simulink model "SystemModel"  (Simulink 8.6)
settings: Solver=ode45  StartTime=0.0  StopTime=25  RelTol=1e-3
undefined symbols (not defined in the file): Alt, altSaturation, ControlDriverGain, CurrentDriverBias, mBackEMF, mDrag, mElecDynDen, mElecDynNum, mHeliDynDen, mHeliDynNum, mLiftTorque, mMechDynDen, mMechDynNum, mPID, mSat, mTConst, potentiometerBias, potentiometerGain, RadPerDeg, tBackEMF, tElecDynDen, tElecDynNum, tHeliDynDen, tHeliDynNum, tMechDynDen, tMechDynNum, torqueFromAltMotorMass, torqueFromYawMotorMass, tPID, tSat, tTConst, tTorque, Yaw, yawSaturation
libraries: simulink x4, simulink_extras x1
settings Model: Creator=Leos  LastModifiedBy=Wyatt
settings DataIOCC: LimitDataPoints=off
settings DebuggingCC: ParameterTunabilityLossMsg=error  FcnCallInpInsideContextMsg=UseLocalSettings
settings ConfigComp: CovSFcnEnable=off

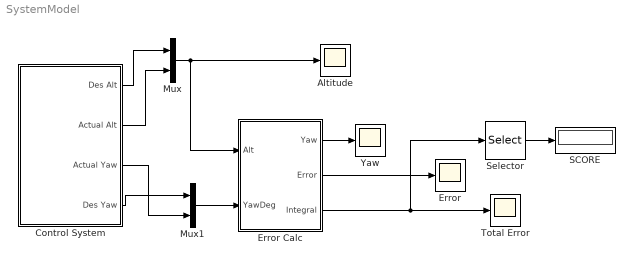
== system SystemModel ==
  Altitude : Scope
  Control System : Subsystem
  Error : Scope
  Error Calc : Subsystem
  Mux : Mux  Inputs=2
  Mux1 : Mux  Inputs=2
  SCORE : Display
  Selector : Selector  InputPortWidth=3  IndexOptions=Index vector (dialog)  Indices=[3]  OutputSizes=1
  Total Error : Scope
  Yaw : Scope
  wires:
  Mux/1 -> Error Calc/1(Alt), Altitude/1
  Control System/1(Des Alt) -> Mux/1
  Control System/2(Actual Alt) -> Mux/2
  Control System/3(Actual Yaw) -> Mux1/2
  Control System/4(Des Yaw) -> Mux1/1
  Mux1/1 -> Error Calc/2(YawDeg)
  Error Calc/1(Yaw) -> Yaw/1
  Error Calc/2(Error) -> Error/1
  Error Calc/3(Integral) -> Selector/1, Total Error/1
  Selector/1 -> SCORE/1

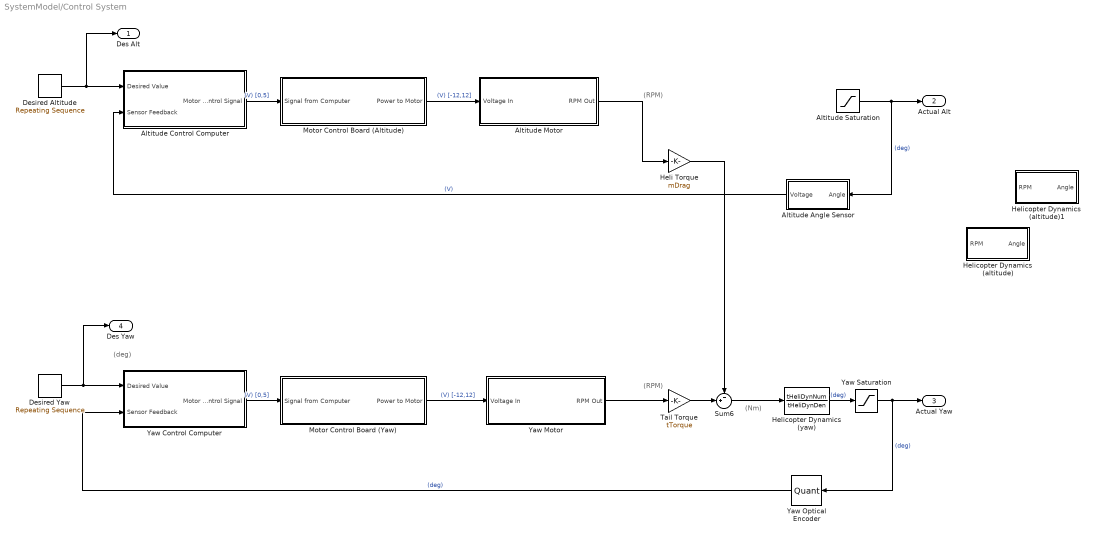
== system SystemModel/Control System ==
  note: (RPM)
  note: (deg)
  note: (RPM)
  note: (Nm)
  Altitude Saturation : Saturate  UpperLimit=altSaturation  LowerLimit=-altSaturation
  Altitude Angle Sensor : Subsystem
  Altitude Control Computer : Subsystem
  Altitude Motor : Subsystem
  Desired Altitude : simulink/Sources/Repeating Sequence  rep_seq_t=Alt(2,:)  rep_seq_y=Alt(1,:)
  Desired Yaw : simulink/Sources/Repeating Sequence  rep_seq_t=Yaw(2,:)  rep_seq_y=Yaw(1,:)
  Heli Torque : Gain  Gain=mDrag
  Helicopter Dynamics (yaw) : TransferFcn  Numerator=tHeliDynNum  Denominator=tHeliDynDen
  Helicopter Dynamics (altitude) : Subsystem
  Helicopter Dynamics (altitude)1 : Subsystem
  Motor Control Board (Altitude) : Subsystem
  Motor Control Board (Yaw) : Subsystem
  Sum6 : Sum  Inputs=-+|
  Tail Torque : Gain  Gain=tTorque
  Yaw Saturation : Saturate  UpperLimit=yawSaturation  LowerLimit=0
  Yaw Control Computer : Subsystem
  Yaw Motor : Subsystem
  Yaw Optical Encoder : Quantizer  QuantizationInterval=yawEncoderQuantization
  Des Alt : Outport
  Actual Alt : Outport  Port=2
  Actual Yaw : Outport  Port=3
  Des Yaw : Outport  Port=4
  wires:
  Desired Altitude/1 -> Altitude Control Computer/1(Desired Value), Des Alt/1
  Helicopter Dynamics (yaw)/1 -> Yaw Saturation/1  "(deg)"
  Desired Yaw/1 -> Yaw Control Computer/1(Desired Value), Des Yaw/1
  Altitude Motor/1(RPM Out) -> Heli Torque/1
  Yaw Optical Encoder/1 -> Yaw Control Computer/2(Sensor Feedback)  "(deg)"
  Yaw Control Computer/1(Motor Driver Control Signal) -> Motor Control Board (Yaw)/1(Signal from Computer)  "(V) [0,5]"
  Altitude Control Computer/1(Motor Driver Control Signal) -> Motor Control Board (Altitude)/1(Signal from Computer)  "(V) [0,5]"
  Motor Control Board (Altitude)/1(Power to Motor) -> Altitude Motor/1(Voltage In)  "(V) [-12,12]"
  Motor Control Board (Yaw)/1(Power to Motor) -> Yaw Motor/1(Voltage In)  "(V) [-12,12]"
  Yaw Motor/1(RPM Out) -> Tail Torque/1
  Altitude Angle Sensor/1(Voltage) -> Altitude Control Computer/2(Sensor Feedback)  "(V)"
  Altitude Saturation/1 -> Actual Alt/1, Altitude Angle Sensor/1(Angle)  "(deg)"
  Yaw Saturation/1 -> Yaw Optical Encoder/1, Actual Yaw/1  "(deg)"
  Tail Torque/1 -> Sum6/2
  Sum6/1 -> Helicopter Dynamics (yaw)/1
  Heli Torque/1 -> Sum6/1

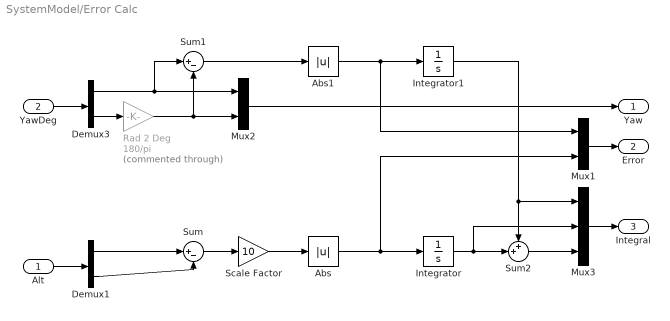
== system SystemModel/Error Calc ==
  Alt : Inport
  YawDeg : Inport  Port=2
  Abs : Abs
  Abs1 : Abs
  Demux1 : Demux  Outputs=2
  Demux3 : Demux  Outputs=2
  Integrator : Integrator
  Integrator1 : Integrator
  Mux1 : Mux  Inputs=2
  Mux2 : Mux  Inputs=2
  Mux3 : Mux  Inputs=3
  Rad 2 Deg : Gain  Commented=through  Gain=180/pi
  Scale Factor : Gain  Gain=10
  Sum : Sum  Inputs=|+-
  Sum1 : Sum  Inputs=|+-
  Sum2 : Sum  Inputs=++|
  Yaw : Outport
  Error : Outport  Port=2
  Integral : Outport  Port=3
  wires:
  YawDeg/1 -> Demux3/1
  Alt/1 -> Demux1/1
  Mux2/1 -> Yaw/1
  Rad 2 Deg/1 -> Sum1/2, Mux2/2
  Demux3/2 -> Rad 2 Deg/1
  Demux3/1 -> Sum1/1, Mux2/1
  Demux1/1 -> Sum/1
  Demux1/2 -> Sum/2
  Sum/1 -> Scale Factor/1
  Mux1/1 -> Error/1
  Sum1/1 -> Abs1/1
  Abs1/1 -> Mux1/1, Integrator1/1
  Scale Factor/1 -> Abs/1
  Abs/1 -> Mux1/2, Integrator/1
  Mux3/1 -> Integral/1
  Integrator/1 -> Mux3/2, Sum2/2
  Integrator1/1 -> Mux3/1, Sum2/1
  Sum2/1 -> Mux3/3

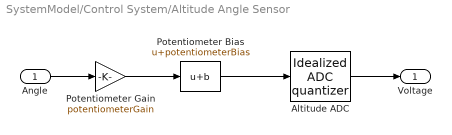
== system SystemModel/Control System/Altitude Angle Sensor ==
  Angle : Inport
  Altitude ADC : simulink_extras/Additional Discrete/Idealized ADC quantizer  NumberOfConverterBits=ADC_bitwidth  Vmin=ground  Vmax=Vss  OutputDataType=int16  OutputNegativeValues=off
  Potentiometer Bias : Bias  Bias=potentiometerBias
  Potentiometer Gain : Gain  Gain=potentiometerGain
  Voltage : Outport
  wires:
  Potentiometer Bias/1 -> Altitude ADC/1
  Angle/1 -> Potentiometer Gain/1
  Potentiometer Gain/1 -> Potentiometer Bias/1
  Altitude ADC/1 -> Voltage/1

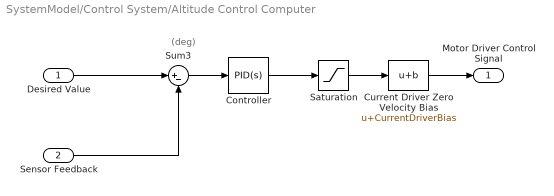
== system SystemModel/Control System/Altitude Control Computer ==
  note: (deg)
  Desired Value : Inport
  Sensor Feedback : Inport  Port=2
  Controller : simulink/Continuous/PID Controller  Controller=PID  TimeDomain=Continuous-time  SampleTime=-1  IntegratorMethod=Forward Euler  FilterMethod=Forward Euler  Form=Parallel  UseFilter=on  ControllerParametersSource=internal  P=mPID(1)  I=mPID(2)  D=mPID(3)  N=100  InitialConditionSource=internal  InitialConditionForIntegrator=0  InitialConditionForFilter=0  ExternalReset=none  LimitOutput=off  UpperSaturationLimit=inf  LowerSaturationLimit=-inf  LinearizeAsGain=on  AntiWindupMode=none  Kb=1  TrackingMode=off  Kt=1  PParamMin=[]  PParamMax=[]  IParamMin=[]  IParamMax=[]  DParamMin=[]  DParamMax=[]  NParamMin=[]  NParamMax=[]  KbParamMin=[]  KbParamMax=[]  KtParamMin=[]  KtParamMax=[]  POutMin=[]  POutMax=[]  IOutMin=[]  IOutMax=[]  DOutMin=[]  DOutMax=[]  NOutMin=[]  NOutMax=[]  KbOutMin=[]  KbOutMax=[]  KtOutMin=[]  KtOutMax=[]  IntegratorOutMin=[]  IntegratorOutMax=[]  FilterOutMin=[]  FilterOutMax=[]  SumOutMin=[]  SumOutMax=[]  SumI1OutMin=[]  SumI1OutMax=[]  SumI2OutMin=[]  SumI2OutMax=[]  SumI3OutMin=[]  SumI3OutMax=[]  SumDOutMin=[]  SumDOutMax=[]  SaturationOutMin=[]  SaturationOutMax=[]  IntegratorContinuousStateAttributes=''  IntegratorStateMustResolveToSignalObject=off  IntegratorRTWStateStorageClass=Auto  FilterContinuousStateAttributes=''  FilterStateMustResolveToSignalObject=off  FilterRTWStateStorageClass=Auto  DifferentiatorICPrevScaledInput=0  DifferentiatorOutMin=[]  DifferentiatorOutMax=[]
  Current Driver Zero Velocity Bias : Bias  Bias=CurrentDriverBias
  Saturation : Saturate  UpperLimit=mSat  LowerLimit=-mSat
  Sum3 : Sum  Inputs=|+-
  Motor Driver Control Signal : Outport
  wires:
  Desired Value/1 -> Sum3/1
  Sensor Feedback/1 -> Sum3/2
  Sum3/1 -> Controller/1
  Saturation/1 -> Current Driver Zero Velocity Bias/1
  Controller/1 -> Saturation/1
  Current Driver Zero Velocity Bias/1 -> Motor Driver Control Signal/1

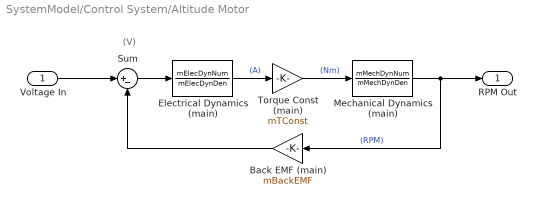
== system SystemModel/Control System/Altitude Motor ==
  note: (V)
  Voltage In : Inport
  Back EMF (main) : Gain  Gain=mBackEMF
  Electrical Dynamics (main) : TransferFcn  Numerator=mElecDynNum  Denominator=mElecDynDen
  Mechanical Dynamics (main) : TransferFcn  Numerator=mMechDynNum  Denominator=mMechDynDen
  Sum : Sum  Inputs=|+-
  Torque Const (main) : Gain  Gain=mTConst
  RPM Out : Outport
  wires:
  Voltage In/1 -> Sum/1
  Torque Const (main)/1 -> Mechanical Dynamics (main)/1  "(Nm)"
  Back EMF (main)/1 -> Sum/2
  Mechanical Dynamics (main)/1 -> RPM Out/1, Back EMF (main)/1  "(RPM)"
  Electrical Dynamics (main)/1 -> Torque Const (main)/1  "(A)"
  Sum/1 -> Electrical Dynamics (main)/1

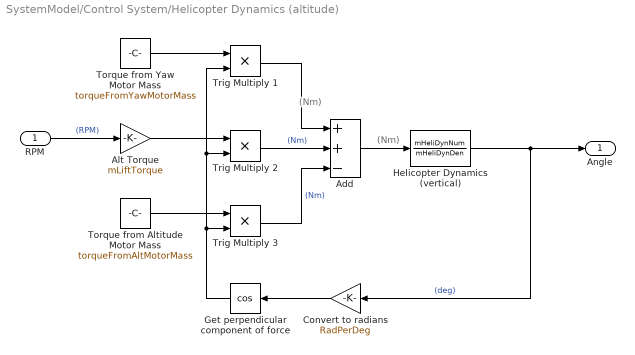
== system SystemModel/Control System/Helicopter Dynamics (altitude) ==
  note: (Nm)
  note: (Nm)
  RPM : Inport
  Add : Sum  Inputs=++-
  Alt Torque : Gain  Gain=mLiftTorque
  Convert to radians : Gain  Gain=RadPerDeg
  Get perpendicular component of force : Trigonometry  Operator=cos
  Helicopter Dynamics (vertical) : TransferFcn  Numerator=mHeliDynNum  Denominator=mHeliDynDen
  Torque from Altitude Motor Mass : Constant  Value=torqueFromAltMotorMass
  "Torque from Yaw Motor Mass " : Constant  Value=torqueFromYawMotorMass
  Trig Multiply 1 : Product
  Trig Multiply 2 : Product
  Trig Multiply 3 : Product
  Angle : Outport
  wires:
  RPM/1 -> Alt Torque/1  "(RPM)"
  Helicopter Dynamics (vertical)/1 -> Angle/1, Convert to radians/1  "(deg)"
  Alt Torque/1 -> Trig Multiply 2/1
  Get perpendicular component of force/1 -> Trig Multiply 3/2, Trig Multiply 2/2, Trig Multiply 1/2
  "Torque from Yaw Motor Mass "/1 -> Trig Multiply 1/1
  Add/1 -> Helicopter Dynamics (vertical)/1
  Trig Multiply 2/1 -> Add/2  "(Nm)"
  Trig Multiply 1/1 -> Add/1
  Torque from Altitude Motor Mass/1 -> Trig Multiply 3/1
  Trig Multiply 3/1 -> Add/3  "(Nm)"
  Convert to radians/1 -> Get perpendicular component of force/1

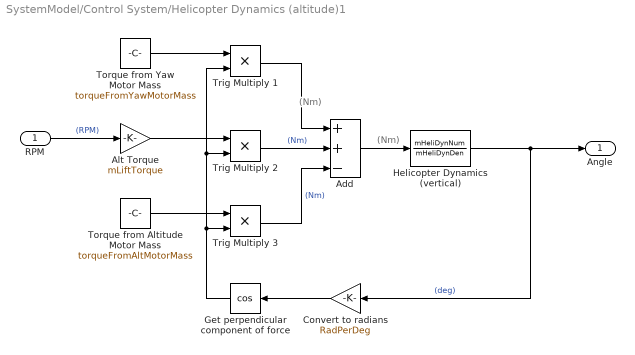
== system SystemModel/Control System/Helicopter Dynamics (altitude)1 ==
  note: (Nm)
  note: (Nm)
  RPM : Inport
  Add : Sum  Inputs=++-
  Alt Torque : Gain  Gain=mLiftTorque
  Convert to radians : Gain  Gain=RadPerDeg
  Get perpendicular component of force : Trigonometry  Operator=cos
  Helicopter Dynamics (vertical) : TransferFcn  Numerator=mHeliDynNum  Denominator=mHeliDynDen
  Torque from Altitude Motor Mass : Constant  Value=torqueFromAltMotorMass
  "Torque from Yaw Motor Mass " : Constant  Value=torqueFromYawMotorMass
  Trig Multiply 1 : Product
  Trig Multiply 2 : Product
  Trig Multiply 3 : Product
  Angle : Outport
  wires:
  Convert to radians/1 -> Get perpendicular component of force/1
  Trig Multiply 3/1 -> Add/3  "(Nm)"
  Torque from Altitude Motor Mass/1 -> Trig Multiply 3/1
  Trig Multiply 1/1 -> Add/1
  Trig Multiply 2/1 -> Add/2  "(Nm)"
  Add/1 -> Helicopter Dynamics (vertical)/1
  "Torque from Yaw Motor Mass "/1 -> Trig Multiply 1/1
  Get perpendicular component of force/1 -> Trig Multiply 1/2, Trig Multiply 2/2, Trig Multiply 3/2
  Alt Torque/1 -> Trig Multiply 2/1
  Helicopter Dynamics (vertical)/1 -> Convert to radians/1, Angle/1  "(deg)"
  RPM/1 -> Alt Torque/1  "(RPM)"

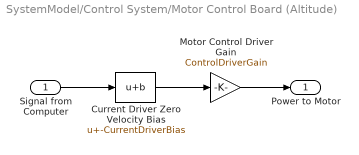
== system SystemModel/Control System/Motor Control Board (Altitude) ==
  Signal from Computer : Inport
  Current Driver Zero Velocity Bias : Bias  Bias=-CurrentDriverBias
  Motor Control Driver Gain : Gain  Gain=ControlDriverGain
  Power to Motor : Outport
  wires:
  Motor Control Driver Gain/1 -> Power to Motor/1
  Signal from Computer/1 -> Current Driver Zero Velocity Bias/1
  Current Driver Zero Velocity Bias/1 -> Motor Control Driver Gain/1

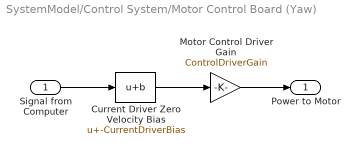
== system SystemModel/Control System/Motor Control Board (Yaw) ==
  Signal from Computer : Inport
  Current Driver Zero Velocity Bias : Bias  Bias=-CurrentDriverBias
  Motor Control Driver Gain : Gain  Gain=ControlDriverGain
  Power to Motor : Outport
  wires:
  Motor Control Driver Gain/1 -> Power to Motor/1
  Signal from Computer/1 -> Current Driver Zero Velocity Bias/1
  Current Driver Zero Velocity Bias/1 -> Motor Control Driver Gain/1

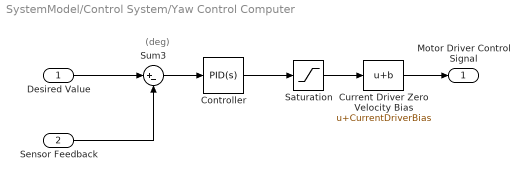
== system SystemModel/Control System/Yaw Control Computer ==
  note: (deg)
  Desired Value : Inport
  Sensor Feedback : Inport  Port=2
  Controller : simulink/Continuous/PID Controller  Controller=PID  TimeDomain=Continuous-time  SampleTime=-1  IntegratorMethod=Forward Euler  FilterMethod=Forward Euler  Form=Parallel  UseFilter=on  ControllerParametersSource=internal  P=tPID(1)  I=tPID(2)  D=tPID(3)  N=100  InitialConditionSource=internal  InitialConditionForIntegrator=0  InitialConditionForFilter=0  ExternalReset=none  LimitOutput=off  UpperSaturationLimit=inf  LowerSaturationLimit=-inf  LinearizeAsGain=on  AntiWindupMode=none  Kb=1  TrackingMode=off  Kt=1  PParamMin=[]  PParamMax=[]  IParamMin=[]  IParamMax=[]  DParamMin=[]  DParamMax=[]  NParamMin=[]  NParamMax=[]  KbParamMin=[]  KbParamMax=[]  KtParamMin=[]  KtParamMax=[]  POutMin=[]  POutMax=[]  IOutMin=[]  IOutMax=[]  DOutMin=[]  DOutMax=[]  NOutMin=[]  NOutMax=[]  KbOutMin=[]  KbOutMax=[]  KtOutMin=[]  KtOutMax=[]  IntegratorOutMin=[]  IntegratorOutMax=[]  FilterOutMin=[]  FilterOutMax=[]  SumOutMin=[]  SumOutMax=[]  SumI1OutMin=[]  SumI1OutMax=[]  SumI2OutMin=[]  SumI2OutMax=[]  SumI3OutMin=[]  SumI3OutMax=[]  SumDOutMin=[]  SumDOutMax=[]  SaturationOutMin=[]  SaturationOutMax=[]  IntegratorContinuousStateAttributes=''  IntegratorStateMustResolveToSignalObject=off  IntegratorRTWStateStorageClass=Auto  FilterContinuousStateAttributes=''  FilterStateMustResolveToSignalObject=off  FilterRTWStateStorageClass=Auto  DifferentiatorICPrevScaledInput=0  DifferentiatorOutMin=[]  DifferentiatorOutMax=[]
  Current Driver Zero Velocity Bias : Bias  Bias=CurrentDriverBias
  Saturation : Saturate  UpperLimit=tSat  LowerLimit=-tSat
  Sum3 : Sum  Inputs=|+-
  Motor Driver Control Signal : Outport
  wires:
  Desired Value/1 -> Sum3/1
  Sensor Feedback/1 -> Sum3/2
  Sum3/1 -> Controller/1
  Saturation/1 -> Current Driver Zero Velocity Bias/1
  Controller/1 -> Saturation/1
  Current Driver Zero Velocity Bias/1 -> Motor Driver Control Signal/1

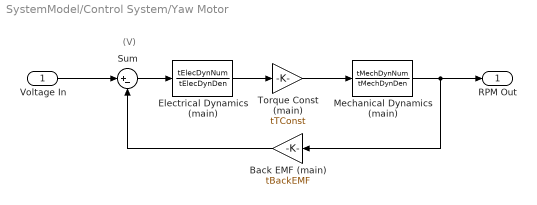
== system SystemModel/Control System/Yaw Motor ==
  note: (V)
  Voltage In : Inport
  Back EMF (main) : Gain  Gain=tBackEMF
  Electrical Dynamics (main) : TransferFcn  Numerator=tElecDynNum  Denominator=tElecDynDen
  Mechanical Dynamics (main) : TransferFcn  Numerator=tMechDynNum  Denominator=tMechDynDen
  Sum : Sum  Inputs=|+-
  Torque Const (main) : Gain  Gain=tTConst
  RPM Out : Outport
  wires:
  Voltage In/1 -> Sum/1
  Torque Const (main)/1 -> Mechanical Dynamics (main)/1
  Back EMF (main)/1 -> Sum/2
  Mechanical Dynamics (main)/1 -> RPM Out/1, Back EMF (main)/1
  Electrical Dynamics (main)/1 -> Torque Const (main)/1
  Sum/1 -> Electrical Dynamics (main)/1
